simulink model "doc_iterative_decoding_sccc"  (R2014a)
settings: Solver=ode45  SolverMode=SingleTasking  StartTime=0.0  StopTime=500  RelTol=1e-3
PostLoadFcn:
  | commsccc_setup;
undefined symbols (not defined in the file or in its folder): Max, SCCC_len, SCCC_numIter, SCCC_Var
libraries: commcnvcod2 x4, commblkintrlv2 x3, commchan3 x1, commrandsrc2 x1, dspsigops x1, commsink2 x1, dspstat3 x1, dspsrcs4 x1, commutil2 x1
CloseFcn:
  | clear SCCC_EbN0dB SCCC_R SCCC_Var SCCC_len SCCC_numIter SCCC_seed SCCC_trellis1 SCCC_trellis2 scccSigsOut
Description:
  | Iterative Decoding of a Serially Concatenated Convolutional Code (SCCC)
settings Model: CovMetricSettings=d  ExtModeAutoUpdateStatusClock=off  Creator=The MathWorks Inc.
settings SolverCC: ZeroCrossControl=DisableAll
settings DataIOCC: LimitDataPoints=off  SignalLoggingSaveFormat=ModelDataLogs  SaveOutput=off  SaveTime=off  SignalLoggingName=scccSigsOut
settings OptimizationCC: BlockReduction=off  InlineParams=on  InlineInvariantSignals=on  ExpressionDepthLimit=2147483647  InitFltsAndDblsToZero=on  EfficientMapNaN2IntZero=off
settings DebuggingCC: SaveWithParameterizedLinksMsg=none  UnderspecifiedInitializationDetection=Classic  CheckExecutionContextPreStartOutputMsg=on  CheckExecutionContextRuntimeOutputMsg=on  SignalResolutionControl=TryResolveAllWithWarning  SolverPrmCheckMsg=none  MultiTaskDSMMsg=warning  MultiTaskCondExecSysMsg=none  SigSpecEnsureSampleTimeMsg=none  FcnCallInpInsideContextMsg=UseLocalSettings  StateNameClashWarn=warning
settings HardwareCC: TargetUnknown=on
settings RTWCC: IncludeERTFirstTime=on
settings GRTTargetCC: TargetFcnLib=ansi_tfl_tmw.mat  CombineOutputUpdateFcns=off  GRTInterface=on

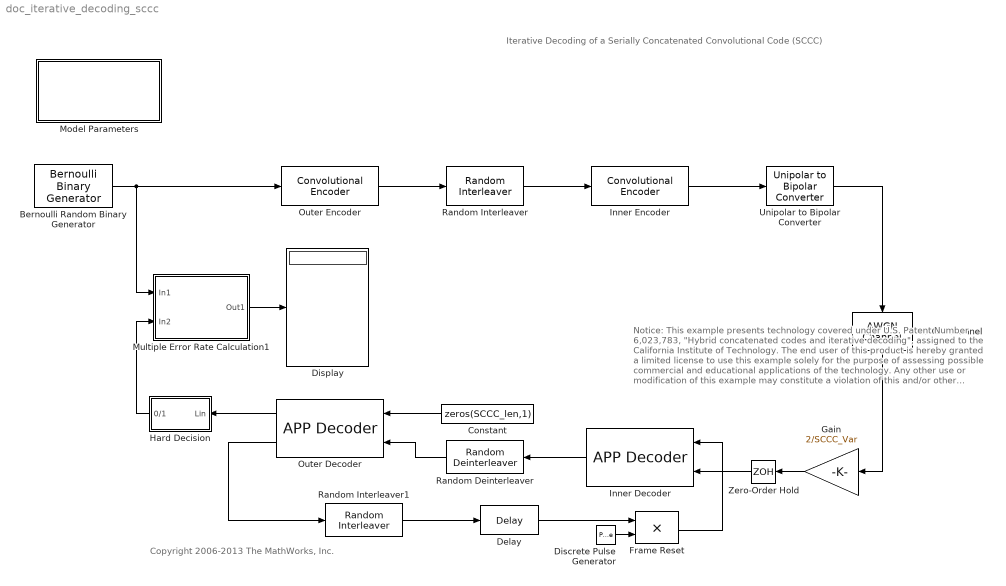
== system doc_iterative_decoding_sccc ==
  note: Notice: This example presents technology
      | covered under U.S. Patent Number 6,023,783,
      | "Hybrid concatenated codes and iterative decoding",
      | assigned to the California Institute of Technology.
      |
      | The end user of this product is hereby granted a limited license
      | to use this example solely for the purpose of  assessing
      | possible commercial and educational applications of the
      | technology. Any other use or modification of this example
      | may constitute a violation of this and/or other patents.
  note: Iterative Decoding of a Serially Concatenated Convolutional Code (SCCC)
  note: Copyright 2006-2013 The MathWorks, Inc.
  AWGN Channel : commchan3/AWGN Channel  InputProcessing=Columns as channels (frame based)  seed=123449  noiseMode=Variance from mask  EbNodB=10  EsNodB=0  SNRdB=10  bitsPerSym=1  Ps=1  Tsym=1/len/3  variance=SCCC_Var
  Bernoulli Random Binary Generator : commrandsrc2/Bernoulli Binary Generator  P=0.5  seed=12343  Ts=SCCC_numIter/SCCC_len  frameBased=on  sampPerFrame=SCCC_len  orient=off  outDataType=boolean
  Constant : Constant  Value=zeros(SCCC_len,1)  VectorParams1D=off  FramePeriod=1
      settings: SamplingMode=Frame based
  Delay : dspsigops/Delay  InputProcessing=Columns as channels (frame based)  dly_unit=Samples  delay=SCCC_len*2  ic_detail=off  dif_ic_for_ch=off  dif_ic_for_dly=off  ic=0  reset_popup=None
  Discrete Pulse Generator : DiscretePulseGenerator  Period=SCCC_numIter  PulseWidth=SCCC_numIter-1  PhaseDelay=1
  Display : Display
  Frame Reset : Product  SaturateOnIntegerOverflow=on  InputSameDT=on  OutDataTypeStr=Inherit: Same as first input
  Gain : Gain  Gain=2/SCCC_Var  SaturateOnIntegerOverflow=on  OutDataTypeStr=Inherit: Same as input  ParamDataTypeStr=Inherit: Same as input
  Hard Decision : Subsystem  mask(Hard Decision){}
      mask help: Likelihood to binary transformation.
  Inner Decoder : commcnvcod2/APP Decoder  trellis=poly2trellis([3 3],[7 0 5;0 7 6],[7 7])  termMethod=Truncated  algorithm=Max*  maxStarNumScaleBits=3  disableLcOut=on
  Inner Encoder : commcnvcod2/Convolutional Encoder  trellis=poly2trellis([3 3],[7 0 5;0 7 6],[7 7])  opMode=Truncated (reset every frame)  DelayedResetAction=off  hasIniStPort=off  hasFinStPort=off  usePuncVector=off  punctureVector=[1; 1; 0; 1; 0; 1]  reset=Unused parameter value
  Model Parameters : Subsystem  mask(Model Parameters){SCCC_EbN0dB=1.5, SCCC_len=1024, SCCC_numIter=6, SCCC_seed=19046}
      mask prompts: SCCC_EbN0dB "Eb/No:"; SCCC_len "Block size:"; SCCC_numIter "Number of iterations:"; SCCC_seed "Seed:"
      mask help: Load model parameters in MATLAB workspace.
      mask init:
      | commsccc_setup;
      mask Help: helpview(commdhelp);
      mask Callback SCCC_EbN0dB: commsccc_setup
      mask Callback SCCC_len: commsccc_setup
      mask Callback SCCC_numIter: commsccc_setup
      mask Callback SCCC_seed: commsccc_setup
      mask Display:
      | disp(['Eb/No   ' num2str(SCCC_EbN0dB,'%3.1f') 'dB' ...
      | sprintf('\n') 'Block size   ' num2str(SCCC_len,'%7.0f') ...
      | sprintf('\n') 'Iterations   ' num2str(SCCC_numIter,'%3.0f')  ...
      | sprintf('\n') 'Seed   ' num2str(SCCC_seed,'%7.0f')])
  Multiple Error Rate Calculation1 : Subsystem
      mask Display: disp('Multiple\nIteration\nError Rate\nCalculation')
  Outer Decoder : commcnvcod2/APP Decoder  trellis=poly2trellis(3, [7 5],7)  termMethod=Truncated  algorithm=Max*  maxStarNumScaleBits=3  disableLcOut=off
  Outer Encoder : commcnvcod2/Convolutional Encoder  trellis=poly2trellis(3, [7 5],7)  opMode=Truncated (reset every frame)  DelayedResetAction=off  hasIniStPort=off  hasFinStPort=off  usePuncVector=off  punctureVector=[1; 1; 0; 1; 0; 1]  reset=Unused parameter value
  Random Deinterleaver : commblkintrlv2/Random Deinterleaver  N=SCCC_len*2  seed=SCCC_seed
  Random Interleaver : commblkintrlv2/Random Interleaver  N=SCCC_len*2  seed=SCCC_seed
  Random Interleaver1 : commblkintrlv2/Random Interleaver  N=SCCC_len*2  seed=SCCC_seed
  Unipolar to Bipolar Converter : commutil2/Unipolar to Bipolar Converter  M=2  polarity=Positive  dataType=double
  Zero-Order Hold : ZeroOrderHold  SampleTime=SCCC_numIter
  wires:
  AWGN Channel/1 -> Gain/1
  Unipolar to Bipolar Converter/1 -> AWGN Channel/1
  Bernoulli Random Binary Generator/1 -> Multiple Error Rate Calculation1/1(In1), Outer Encoder/1
  Outer Encoder/1 -> Random Interleaver/1
  Random Interleaver/1 -> Inner Encoder/1
  Inner Encoder/1 -> Unipolar to Bipolar Converter/1
  Inner Decoder/1 -> Random Deinterleaver/1
  Random Deinterleaver/1 -> Outer Decoder/2
  Outer Decoder/2 -> Random Interleaver1/1
  Constant/1 -> Outer Decoder/1
  Frame Reset/1 -> Inner Decoder/1
  Random Interleaver1/1 -> Delay/1
  Outer Decoder/1 -> Hard Decision/1(Lin)
  Hard Decision/1(0/1) -> Multiple Error Rate Calculation1/2(In2)
  Multiple Error Rate Calculation1/1(Out1) -> Display/1
  Gain/1 -> Zero-Order Hold/1
  Discrete Pulse Generator/1 -> Frame Reset/2
  Delay/1 -> Frame Reset/1
  Zero-Order Hold/1 -> Inner Decoder/2

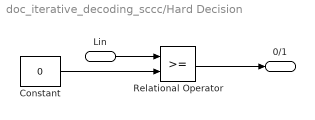
== system doc_iterative_decoding_sccc/Hard Decision ==
  Lin : Inport
  Constant : Constant  Value=0
  Relational Operator : RelationalOperator  InputSameDT=on
  0/1 : Outport
  wires:
  Relational Operator/1 -> 0/1/1
  Lin/1 -> Relational Operator/1
  Constant/1 -> Relational Operator/2

== system doc_iterative_decoding_sccc/Model Parameters ==

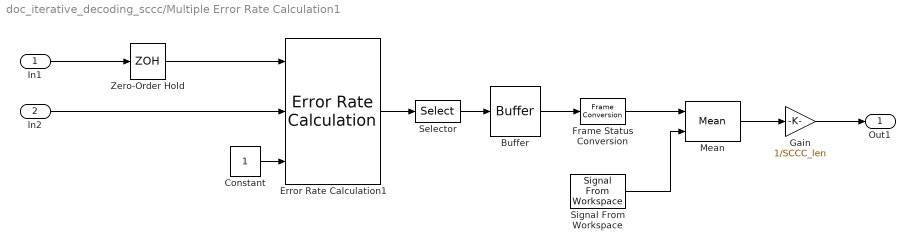
== system doc_iterative_decoding_sccc/Multiple Error Rate Calculation1 ==
  In1 : Inport
  In2 : Inport  Port=2
  Buffer : Buffer  N=SCCC_numIter  TreatMby1Signals=One channel
  Constant : Constant
  Error Rate Calculation1 : commsink2/Error Rate Calculation  N=0  st_delay=0  cp_mode=Entire frame  subframe=[]  PMode=Port  WsName=ErrorVec1  RsMode2=on  stop=off  numErr=100  maxBits=1e6
  Frame Status Conversion : FrameConversion  OutFrame=Sample-based
  Gain : Gain  Gain=1/SCCC_len  SaturateOnIntegerOverflow=on  OutDataTypeStr=Inherit: Same as input  ParamDataTypeStr=Inherit: Same as input
  Mean : dspstat3/Mean  run=on  reset_popup=Non-zero sample  directionMode=Each column  dimension=1  treatSBRowAsCol=on  roiEnable=off  roiType=Rectangles  roiPortion=Entire ROI  roiOutput=Individual statistics for each ROI  roiFlag=off  outputDataTypeStr=Inherit: Same as accumulator  outputLastDataTypeStr=Inherit: Same as accumulator  outputMin=[]  outputMax=[]  roundingMode=Floor  overflowMode=off
  Selector : Selector  InputPortWidth=3  Indices=2
  Signal From Workspace : dspsrcs4/Signal From Workspace  X=[1 1]  Ts=SCCC_numIter  nsamps=1  OutputAfterFinalValue=Setting to zero  ignoreOrWarnInputAndFrameLengths=off
  Zero-Order Hold : ZeroOrderHold
  Out1 : Outport
  wires:
  In1/1 -> Zero-Order Hold/1
  Error Rate Calculation1/1 -> Selector/1
  Selector/1 -> Buffer/1
  In2/1 -> Error Rate Calculation1/2
  Buffer/1 -> Frame Status Conversion/1
  Frame Status Conversion/1 -> Mean/1
  Zero-Order Hold/1 -> Error Rate Calculation1/1
  Constant/1 -> Error Rate Calculation1/3
  Mean/1 -> Gain/1
  Gain/1 -> Out1/1
  Signal From Workspace/1 -> Mean/2
